simulink model "simulink_sim"  (R2024b)
settings: Solver=ode4  StartTime=0.0  StopTime=10  FixedStep=1  RelTol=1e-3
settings Model: Creator=Aylar  LastModifiedBy=Aylar

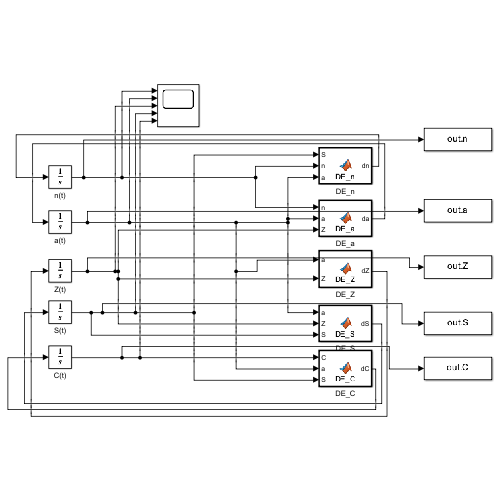
[thumbnail: Simulink's stored preview of the top-level diagram]
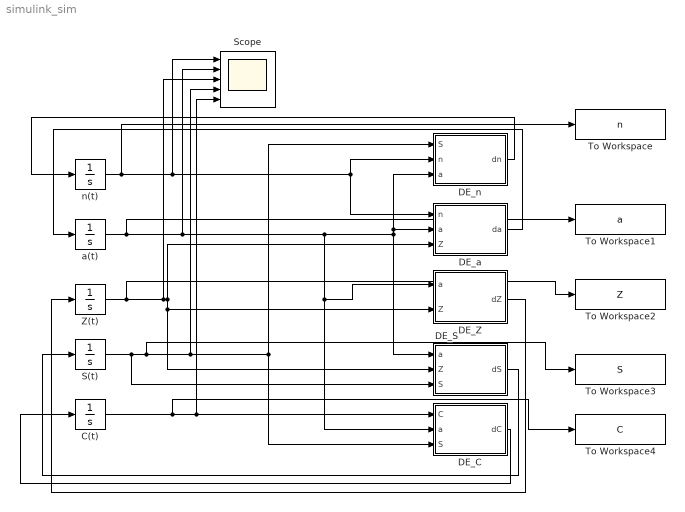
== system simulink_sim ==
  C(t) : Integrator  InitialCondition=0.1
  DE_C : MATLAB Function  TreatAsAtomicUnit=on
  DE_S : MATLAB Function  TreatAsAtomicUnit=on
  DE_Z : MATLAB Function  TreatAsAtomicUnit=on
  DE_a : MATLAB Function  TreatAsAtomicUnit=on
  DE_n : MATLAB Function  TreatAsAtomicUnit=on
  S(t) : Integrator  InitialCondition=0.1
  Scope : Scope  NumInputPorts=5
  To Workspace : ToWorkspace  VariableName=n  SampleTime=-1
      settings: Save2DSignal=2-D array (concatenate along first dimension)
  To Workspace1 : ToWorkspace  VariableName=a  SampleTime=-1
      settings: Save2DSignal=2-D array (concatenate along first dimension)
  To Workspace2 : ToWorkspace  VariableName=Z  SampleTime=-1
      settings: Save2DSignal=2-D array (concatenate along first dimension)
  To Workspace3 : ToWorkspace  VariableName=S  SampleTime=-1
      settings: Save2DSignal=2-D array (concatenate along first dimension)
  To Workspace4 : ToWorkspace  VariableName=C  SampleTime=-1
      settings: Save2DSignal=2-D array (concatenate along first dimension)
  Z(t) : Integrator  InitialCondition=0.1
  a(t) : Integrator  InitialCondition=0.1
  n(t) : Integrator  InitialCondition=0.1
  wires:
  S(t)/1 -> DE_S/3(S), To Workspace3/1, DE_C/3(S), DE_n/1(S), Scope/4
  n(t)/1 -> DE_a/1(n), DE_n/2(n), Scope/1, To Workspace/1
  a(t)/1 -> To Workspace1/1, DE_n/3(a), DE_a/2(a), DE_S/1(a), DE_C/2(a), DE_Z/1(a), Scope/2
  DE_n/1(dn) -> n(t)/1
  Z(t)/1 -> To Workspace2/1, DE_S/2(Z), DE_Z/2(Z), DE_a/3(Z), Scope/3
  DE_a/1(da) -> a(t)/1
  DE_Z/1(dZ) -> Z(t)/1
  DE_S/1(dS) -> S(t)/1
  C(t)/1 -> To Workspace4/1, Scope/5, DE_C/1(C)
  DE_C/1(dC) -> C(t)/1

== matlab function simulink_sim/DE_a ==
  data: n input; a input; da output; Z input
function da = DE_a(n, a, Z)

%#codegen
persistent q pi0 delta alpha0 beta1 theta1 alpha1 beta10 beta2 theta2 alpha2 beta20 pi1 pi2 qc alpha3 lambda11 delta1

if isempty(q)
s = coder.load('sim_data.mat',  'q', 'pi0', 'delta', 'alpha0', 'beta1', ...
    'theta1', 'alpha1', 'beta10', 'beta2', 'theta2', 'alpha2', ...
    'beta20', 'pi1', 'pi2', 'qc', 'alpha3', 'lambda11', 'delta1');

q = s.q; pi0 = s.pi0; delta = s.delta; alpha0 = s.alpha0; beta1 = s.beta1;
theta1 = s.theta1; alpha1 = s.alpha1; beta10 = s.beta10; beta2 = s.beta2; theta2 = s.theta2; alpha2 = s.alpha2;
beta20 = s.beta20; pi1 = s.pi1; pi2 = s.pi2; qc = s.qc; alpha3 = s.alpha3; lambda11 = s.lambda11; delta1 = s.delta1;
end

da = theta1*beta1*n*a - alpha1*a-beta10*a^2-beta2*a*Z;

== matlab function simulink_sim/DE_n ==
  data: dn output; S input; n input; a input
function dn = DE_n(S, n, a)

%#codegen
persistent q pi0 delta alpha0 beta1 theta1 alpha1 beta10 beta2 theta2 alpha2 beta20 pi1 pi2 qc alpha3 lambda11 delta1

if isempty(q)
s = coder.load('sim_data.mat',  'q', 'pi0', 'delta', 'alpha0', 'beta1', ...
    'theta1', 'alpha1', 'beta10', 'beta2', 'theta2', 'alpha2', ...
    'beta20', 'pi1', 'pi2', 'qc', 'alpha3', 'lambda11', 'delta1');

q = s.q; pi0 = s.pi0; delta = s.delta; alpha0 = s.alpha0; beta1 = s.beta1;
theta1 = s.theta1; alpha1 = s.alpha1; beta10 = s.beta10; beta2 = s.beta2; theta2 = s.theta2; alpha2 = s.alpha2;
beta20 = s.beta20; pi1 = s.pi1; pi2 = s.pi2; qc = s.qc; alpha3 = s.alpha3; lambda11 = s.lambda11; delta1 = s.delta1;
end

dn = q+ pi0*delta*S-alpha0*n-beta1*n*a;

== matlab function simulink_sim/DE_Z ==
  data: a input; dZ output; Z input
function dZ = DE_Z(a, Z)

%#codegen
persistent q pi0 delta alpha0 beta1 theta1 alpha1 beta10 beta2 theta2 alpha2 beta20 pi1 pi2 qc alpha3 lambda11 delta1

if isempty(q)
s = coder.load('sim_data.mat',  'q', 'pi0', 'delta', 'alpha0', 'beta1', ...
    'theta1', 'alpha1', 'beta10', 'beta2', 'theta2', 'alpha2', ...
    'beta20', 'pi1', 'pi2', 'qc', 'alpha3', 'lambda11', 'delta1');

q = s.q; pi0 = s.pi0; delta = s.delta; alpha0 = s.alpha0; beta1 = s.beta1;
theta1 = s.theta1; alpha1 = s.alpha1; beta10 = s.beta10; beta2 = s.beta2; theta2 = s.theta2; alpha2 = s.alpha2;
beta20 = s.beta20; pi1 = s.pi1; pi2 = s.pi2; qc = s.qc; alpha3 = s.alpha3; lambda11 = s.lambda11; delta1 = s.delta1;
end

dZ = theta2*beta2*a*Z - alpha2*Z-beta20*Z^2;

== matlab function simulink_sim/DE_S ==
  data: a input; Z input; S input; dS output
function dS = DE_S(a, Z, S)

%#codegen

persistent q pi0 delta alpha0 beta1 theta1 alpha1 beta10 beta2 theta2 alpha2 beta20 pi1 pi2 qc alpha3 lambda11 delta1

if isempty(q)
s = coder.load('sim_data.mat',  'q', 'pi0', 'delta', 'alpha0', 'beta1', ...
    'theta1', 'alpha1', 'beta10', 'beta2', 'theta2', 'alpha2', ...
    'beta20', 'pi1', 'pi2', 'qc', 'alpha3', 'lambda11', 'delta1');

q = s.q; pi0 = s.pi0; delta = s.delta; alpha0 = s.alpha0; beta1 = s.beta1;
theta1 = s.theta1; alpha1 = s.alpha1; beta10 = s.beta10; beta2 = s.beta2; theta2 = s.theta2; alpha2 = s.alpha2;
beta20 = s.beta20; pi1 = s.pi1; pi2 = s.pi2; qc = s.qc; alpha3 = s.alpha3; lambda11 = s.lambda11; delta1 = s.delta1;
end

dS = pi1*alpha1*a+pi2*alpha2*Z-delta*S;

== matlab function simulink_sim/DE_C ==
  data: C input; a input; S input; dC output
function dC = DE_C(C, a, S)

%#codegen
persistent q pi0 delta alpha0 beta1 theta1 alpha1 beta10 beta2 theta2 alpha2 beta20 pi1 pi2 qc alpha3 lambda11 delta1

if isempty(q)
s = coder.load('sim_data.mat',  'q', 'pi0', 'delta', 'alpha0', 'beta1', ...
    'theta1', 'alpha1', 'beta10', 'beta2', 'theta2', 'alpha2', ...
    'beta20', 'pi1', 'pi2', 'qc', 'alpha3', 'lambda11', 'delta1');

q = s.q; pi0 = s.pi0; delta = s.delta; alpha0 = s.alpha0; beta1 = s.beta1;
theta1 = s.theta1; alpha1 = s.alpha1; beta10 = s.beta10; beta2 = s.beta2; theta2 = s.theta2; alpha2 = s.alpha2;
beta20 = s.beta20; pi1 = s.pi1; pi2 = s.pi2; qc = s.qc; alpha3 = s.alpha3; lambda11 = s.lambda11; delta1 = s.delta1;
end

dC = qc - alpha3*C-lambda11*a-delta1*S;
